simulink model "close_loop_circuit_model_with_discrete_compensator"  (R2023a)
settings: Solver=VariableStepAuto  StartTime=0.0  StopTime=0.01  RelTol=1e-3
undefined symbols (not defined in the file): DiscIntNeverNeededParam
libraries: spsSeriesRLCBranchLib x3, simulink x3, spsDiodeLib x2, spsMosfetLib x2, spsCurrentMeasurementLib x1, spsDCVoltageSourceLib x1, spsMultiWindingTransformerLib x1, spsRMSLib x1, spsVoltageMeasurementLib x1, spspowerguiLib x1
settings Model: Creator=Muzaffar Hussain  LastModifiedBy=Muzaffar Hussain

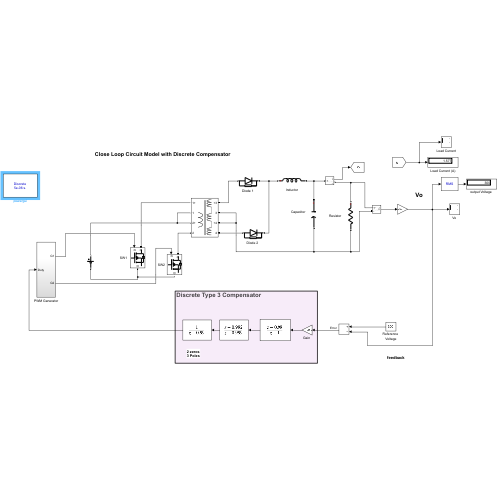
[thumbnail: Simulink's stored preview of the top-level diagram]
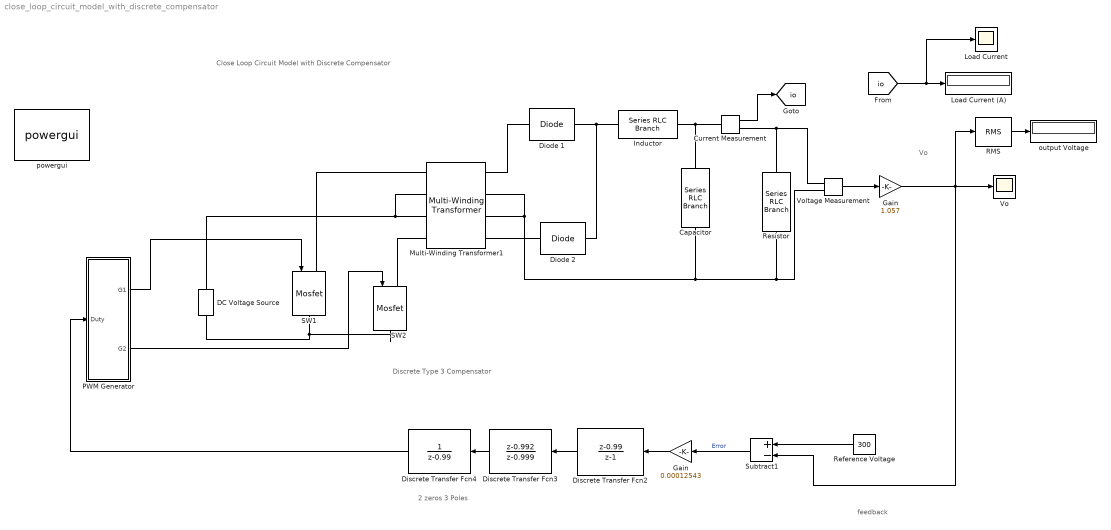
== system close_loop_circuit_model_with_discrete_compensator ==
  note: feedback
  note: Vo
  note: Close Loop Circuit Model with Discrete Compensator
  note: Discrete Type 3 Compensator
  note: 2 zeros
      | 3 Poles
  "Capacitor " : spsSeriesRLCBranchLib/Series RLC Branch  LConnTagsString=__new0  RConnTagsString=__new0  BranchType=C  Resistance=0.33  Inductance=1e-3  SetiL0=off  InitialCurrent=0  Capacitance=33e-6  Setx0=off  InitialVoltage=0  Measurements=None
  Current Measurement : spsCurrentMeasurementLib/Current Measurement  PhasorSimulation=off  OutputType=Complex  PSBequivalent=0
  DC Voltage Source : spsDCVoltageSourceLib/DC Voltage Source  Amplitude=12  Measurements=None
  "Diode 1 " : spsDiodeLib/Diode  Ron=0.1  Lon=0  Vf=0.8  IC=0  UseSnubber=0  Rs=5*10^10  Cs=inf  Measurements=off
  "Diode 2  " : spsDiodeLib/Diode  Ron=0.1  Lon=0  Vf=0.8  IC=0  UseSnubber=0  Rs=5*10^10  Cs=inf  Measurements=off
  Discrete Transfer Fcn2 : DiscreteTransferFcn  Numerator=[1 -0.99]  Denominator=[1 -1]  SampleTime=0.001
  Discrete Transfer Fcn3 : DiscreteTransferFcn  Numerator=[1 -0.992]  Denominator=[1 -0.999]  SampleTime=0.001
  Discrete Transfer Fcn4 : DiscreteTransferFcn  Denominator=[1 -0.99]  SampleTime=0.001
  Gain : Gain  Gain=1.057
  "Gain " : Gain  Gain=0.00012543
  Inductor : spsSeriesRLCBranchLib/Series RLC Branch  LConnTagsString=__new0  RConnTagsString=__new0  BranchType=L  Resistance=0.08  Inductance=2e-3  SetiL0=off  InitialCurrent=0  Capacitance=1e-6  Setx0=off  InitialVoltage=0  Measurements=None
  Load Current : Scope
  Load Current (A) : Display
  Multi-Winding Transformer1 : spsMultiWindingTransformerLib/Multi-Winding Transformer  LeftWindings=2  RightWindings=2  TappedWindings=no taps  NumberOfTaps=0  SetSaturation=off  Hysteresis=off  DataFile='hysteresis.mat'  Measurements=None  UNITS=SI  NominalPower=[500 35000]  NominalVoltages=[12 12 300 300]  WindingResistances=[0.01 0.01 0.001 0.001]  WindingInductances=[0 0 0 0]  Rm=10  Lm=34.4e-03  Saturation=[0 0;4.7956e+10 1.3975e-34;1.9981e+13 1.7703e-34]  SpecifyInitialFlux=off  InitialFlux=0  BreakLoop=off  DiscreteSolver=Trapezoidal iterative  DataType=on  TransfoNumber=1
      settings: LibrarySourceBlock=|
      | sps_lib/Power Grid Elements/Multi-Winding
      | Transformer
  PWM Generator : Subsystem
  RMS : spsRMSLib/RMS  TrueRMS=on  Freq=35E3  RMSInit=0  Ts=0
  Reference Voltage : Constant  Value=300
  "Resistor " : spsSeriesRLCBranchLib/Series RLC Branch  LConnTagsString=__new0  RConnTagsString=__new0  BranchType=R  Resistance=180  Inductance=1e-3  SetiL0=off  InitialCurrent=0  Capacitance=1e-6  Setx0=off  InitialVoltage=0  Measurements=None
  "SW1 " : spsMosfetLib/Mosfet  Ron=0.005  Lon=0  Rd=0.001  Vfd=0  IC=0  Rs=1e6  Cs=inf  Measurements=off
  SW2 : spsMosfetLib/Mosfet  Ron=0.005  Lon=0  Rd=0.001  Vfd=0  IC=0  Rs=1e6  Cs=inf  Measurements=off
  Subtract1 : Sum  Inputs=+-
  "Vo " : Scope
  Voltage Measurement : spsVoltageMeasurementLib/Voltage Measurement  PhasorSimulation=off  OutputType=Complex  PSBequivalent=0
  "output Voltage " : Display
  powergui : spspowerguiLib/powergui  Priority=1  SimulationMode=Discrete  SampleTime=5e-6  frequency=60  Iterations=50  frequencyindice=0  Pbase=100e6  ErrMax=1e-4  UnitsV=kV  UnitsW=MW  buscounter=0  FunctionMessages=off  echomessages=off  EnableUseOfTLC=off  CurrentSourceSwitches=off  DisableSnubberDevices=off  DisableRonSwitches=off  DisableVfSwitches=off  DisplayEquations=off  AutomaticDiscreteSolvers=off  SolverType=Tustin/Backward Euler (TBE)  Interpol=off  ExternalGateDelay=off  methode=off  Ts=100  x0status=blocks  SPID=on  SwTol=0  HookPort=off  NonlinearTolerance=1e-4  nMaxIteration=100  ContinueOnMaxIteration=off  RestoreLinks=warning  ResistiveCurrentMeasurement=off  Frange=[0:2:500]  Ylog=off  Xlog=on  ShowGrid=off  save=off  variable=ZData  structure=0  ZoomFFT=off  StartTime=0.0  cycles=1  DisplayStyle=1  fundamental=60  FreqAxis=off  MaxFrequency=1000  frequencyindicesteady=1  RmsSteady=1  display=off
  tag scope: io=global
  wires:
  PWM Generator/1(G1) -> "SW1 "/1
  PWM Generator/2(G2) -> SW2/1
  Current Measurement/1 -> [io]
  RMS/1 -> "output Voltage "/1
  [io] -> Load Current/1, Load Current (A)/1
  "Gain "/1 -> Discrete Transfer Fcn2/1
  Discrete Transfer Fcn2/1 -> Discrete Transfer Fcn3/1
  Discrete Transfer Fcn3/1 -> Discrete Transfer Fcn4/1
  Subtract1/1 -> "Gain "/1  "Error"
  Reference Voltage/1 -> Subtract1/1
  Discrete Transfer Fcn4/1 -> PWM Generator/1(Duty)
  Gain/1 -> RMS/1, Subtract1/2, "Vo "/1
  Voltage Measurement/1 -> Gain/1
  connections:
  Multi-Winding Transformer1/LConn3 -- DC Voltage Source/RConn1 -- Multi-Winding Transformer1/LConn2
  Voltage Measurement/LConn2 -- "Resistor "/RConn1 -- Multi-Winding Transformer1/RConn3 -- Multi-Winding Transformer1/RConn2 -- "Capacitor "/RConn1
  Voltage Measurement/LConn1 -- "Resistor "/LConn1 -- Current Measurement/RConn1
  DC Voltage Source/LConn1 -- "SW1 "/RConn1 -- SW2/RConn1
  "Diode 2  "/RConn1 -- "Diode 1 "/RConn1 -- Inductor/LConn1
  "Capacitor "/LConn1 -- Current Measurement/LConn1 -- Inductor/RConn1
  Multi-Winding Transformer1/RConn1 -- "Diode 1 "/LConn1
  SW2/LConn1 -- Multi-Winding Transformer1/LConn4
  "Diode 2  "/LConn1 -- Multi-Winding Transformer1/RConn4
  Multi-Winding Transformer1/LConn1 -- "SW1 "/LConn1

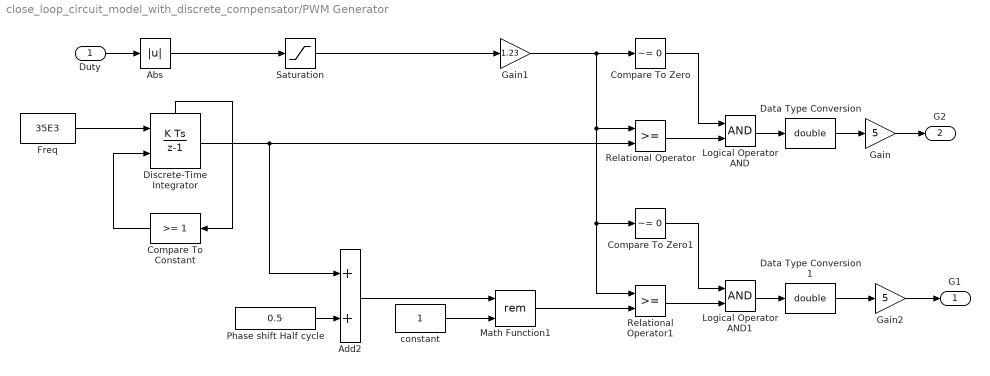
== system close_loop_circuit_model_with_discrete_compensator/PWM Generator ==
  Duty : Inport
  Abs : Abs  SaturateOnIntegerOverflow=off
  Add2 : Sum
  Compare To Constant : simulink/Logic and Bit Operations/Compare To Constant  relop=>=  const=1  OutDataTypeStr=boolean
  Compare To Zero : simulink/Logic and Bit Operations/Compare To Zero  relop=~=  OutDataTypeStr=boolean
  Compare To Zero1 : simulink/Logic and Bit Operations/Compare To Zero  relop=~=  OutDataTypeStr=boolean
  Data Type Conversion : DataTypeConversion  OutDataTypeStr=double  SaturateOnIntegerOverflow=off  RndMeth=Floor
  Data Type Conversion1 : DataTypeConversion  OutDataTypeStr=double  SaturateOnIntegerOverflow=off  RndMeth=Floor
  Discrete-Time Integrator : DiscreteIntegrator  ExternalReset=rising  SampleTime=-1  ShowStatePort=on  ICPrevOutput=DiscIntNeverNeededParam  ICPrevScaledInput=DiscIntNeverNeededParam
  Freq : Constant  Value=35E3  SampleTime=0
  Gain : Gain  Gain=5
  Gain1 : Gain  Gain=1.23
  Gain2 : Gain  Gain=5
  Logical Operator AND : Logic  AllPortsSameDT=off  OutDataTypeStr=boolean
  Logical Operator AND1 : Logic  AllPortsSameDT=off  OutDataTypeStr=boolean
  Math Function1 : Math  Operator=rem  SignedPower=on
  Phase shift Half cycle : Constant  Value=0.5  SampleTime=0
  Relational Operator : RelationalOperator  OutDataTypeStr=boolean  InputSameDT=off
  Relational Operator1 : RelationalOperator  OutDataTypeStr=boolean  InputSameDT=off
  Saturation : Saturate  UpperLimit=0.7  LowerLimit=0.4
  constant : Constant  SampleTime=0
  G1 : Outport  VectorParamsAs1DForOutWhenUnconnected=off
  G2 : Outport  Port=2  VectorParamsAs1DForOutWhenUnconnected=off
  wires:
  Compare To Zero1/1 -> Logical Operator AND1/1
  Compare To Zero/1 -> Logical Operator AND/1
  Relational Operator1/1 -> Logical Operator AND1/2
  Relational Operator/1 -> Logical Operator AND/2
  Phase shift Half cycle/1 -> Add2/2
  Data Type Conversion/1 -> Gain/1
  Data Type Conversion1/1 -> Gain2/1
  Logical Operator AND1/1 -> Data Type Conversion1/1
  Add2/1 -> Math Function1/1
  Math Function1/1 -> Relational Operator1/2
  Logical Operator AND/1 -> Data Type Conversion/1
  constant/1 -> Math Function1/2
  Discrete-Time Integrator/1 -> Relational Operator/2, Add2/1
  Gain1/1 -> Compare To Zero/1, Relational Operator/1, Compare To Zero1/1, Relational Operator1/1
  Freq/1 -> Discrete-Time Integrator/1
  Compare To Constant/1 -> Discrete-Time Integrator/2
  Discrete-Time Integrator/State -> Compare To Constant/1
  Gain/1 -> G2/1
  Gain2/1 -> G1/1
  Abs/1 -> Saturation/1
  Saturation/1 -> Gain1/1
  Duty/1 -> Abs/1
